simulink model "askisi3"  (R2021a)
settings: Solver=VariableStepAuto  StartTime=0.0  StopTime=1  RelTol=1e-3
libraries: spsCurrentMeasurementLib x3, spsVoltageMeasurementLib x3, spsRMSLib x2, spsAsynchronousMachineSIUnitsLib x1, spsNeutralLib x1, spsThreePhaseProgrammableVoltageSourceLib x1, spspowerguiLib x1
settings Model: Creator=up1053646  LastModifiedBy=up1053646

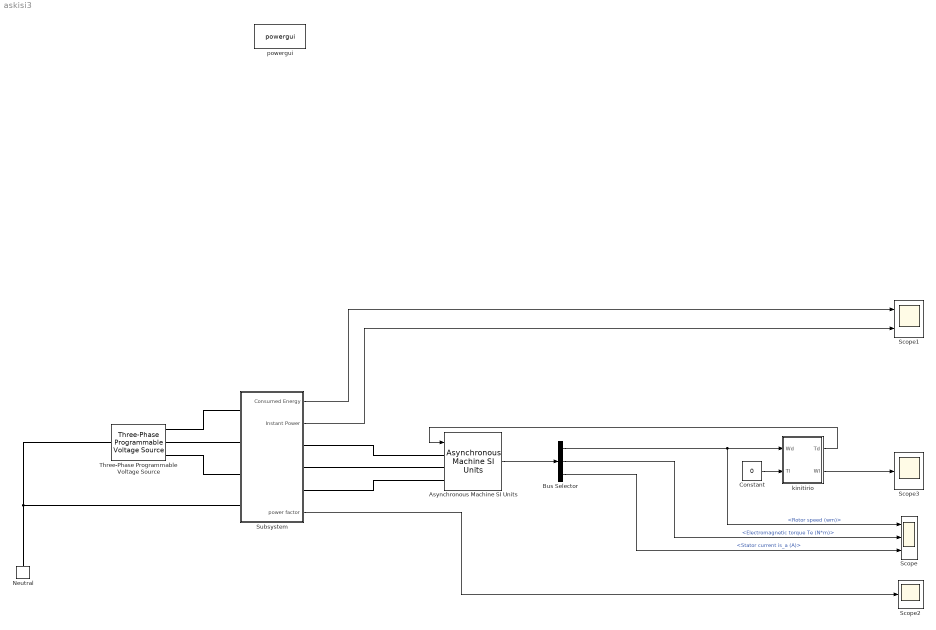
== system askisi3 ==
  Asynchronous Machine SI Units : spsAsynchronousMachineSIUnitsLib/Asynchronous Machine SI Units  RotorType=Squirrel-cage  PresetModel="15:  5.4 HP (4KW)   400 V  50Hz 1430 RPM"  MechanicalLoad=Torque Tm  ShowDetailedParameters=on  ReferenceFrame=Stationary  Units=SI  MeasurementBus=off  NominalParameters=[4000 400 50]  VoltageRatio=1  Stator=[1.405 0.005839]  Rotor=[1.395 0.005839]  Cage1=[0.4155 0.002066]  Cage2=[0.4168 0.0003495]  Lm=0.1722  Mechanical=[0.0131 0.002985 2]  PolePairs=2  InitialConditions=[1 0 0 0 0 0 0 0]  SimulateSaturation=off  Saturation=[14.03593122, 27.81365428, 53.79336849, 72.68890987, 97.98006896, 148.6815601, 215.7428561, 302.9841135, 428.7778367 ; 230, 322, 414, 460, 506, 552, 598, 644, 690]  LoadFlowParameters=1492000  TsPowergui=0  TsBlock=-1  IterativeModel=Trapezoidal non iterative  IterativeDiscreteModel=Trapezoidal non iterative  Pmec=1.492e+006
  Bus Selector : BusSelector  OutputSignals=Mechanical.Rotor speed (wm),Mechanical.Electromagnetic torque Te (N*m),Stator measurements.Stator current is_a (A)
  Constant : Constant  Value=0
  Neutral : spsNeutralLib/Neutral  LConnTagsString=a  NodeNumber=10
      settings: AttributesFormatString=node %<NodeNumber>  SourceProductBaseCode=PS
  Scope : Scope  NumInputPorts=3
  Scope1 : Scope  NumInputPorts=2
  Scope2 : Scope
  Scope3 : Scope
  Subsystem : Subsystem
      settings: PortSchema="{\"entries\":[{\"content\":{\"sides\":[{\"content\":{\"connectorIds\":[\"LConn1\",\"LConn2\",\"LConn3\",\"LConn4\"]},\"type\":\"ConnectorPlacement.EquallySpacedRectSide\",\"uuid\":\"32ddae11-412d-43d8-9429-097a82ad65a8\"},{\"content\":{\"connectorIds\":[\"Out1\",\"Out2\",\"RConn1\",\"RConn2\",\"RConn3\",\"Out3\"],\"side\":\"RIGHT\"},\"type\":\"ConnectorPlacement.EquallySpacedRectSide\",\"uuid\":\"05916abb-9d50-4f55-a81b-b25e6788eafb\"},{\"content\":{\"connectorIds\":[],\"side\":\"TOP\"},\"type\":\"ConnectorPlacement.EquallySpacedRectSide\",\"uuid\":\"ce3b48c4-ab88-427f-b81e-9245e7807eba\"}]},\"type\":\"ConnectorPlacement.EquallySpacedConnector\",\"uuid\":\"fa467998-3027-4402-b2bd-bbf2c58f6d7e\"}],\"packageUris\":[\"http://schema.mathworks.com/mf0/Connector/R2020b\"],\"version\":\"1.0\"}"
  Three-Phase Programmable Voltage Source : spsThreePhaseProgrammableVoltageSourceLib/Three-Phase Programmable Voltage Source  PositiveSequence="[380  0 50]"  VariationEntity=None  VariationType=Table of time-amplitude pairs  VariationTypeAlt=Step  VariationStep=0.5  VariationRate=10  VariationMagnitude=0.3  VariationFrequency=2  VariationTiming=[1 2]  VariationPhaseA=off  Amplitudes=[1 0.8 1.2 1.0]  TimeValues=[0 0.1 0.15 0.2]  HarmonicGeneration=off  HarmonicA=[3 0.2 -25 0]  HarmonicB=[2 0.15 35 2]  Timing="[0.05  3]"  BusType=swing  Pref=0  Qref=0  Qmin=-inf  Qmax=inf
  kinitirio : Subsystem  mask{kin=11000, bin=100, kout=20000, bout=1000, j=0.2, u=2, eff=1}
  powergui : spspowerguiLib/powergui  Priority=1  SimulationMode=Continuous  SampleTime=50e-6  frequency=60  Iterations=50  frequencyindice=50  Pbase=100e6  ErrMax=1e-4  UnitsV=kV  UnitsW=MW  buscounter=0  FunctionMessages=off  echomessages=off  EnableUseOfTLC=off  CurrentSourceSwitches=off  DisableSnubberDevices=off  DisableRonSwitches=off  DisableVfSwitches=off  DisplayEquations=off  AutomaticDiscreteSolvers=off  SolverType=Tustin/Backward Euler (TBE)  Interpol=off  ExternalGateDelay=off  methode=off  Ts=100  x0status=blocks  SPID=on  SwTol=0  HookPort=off  NonlinearTolerance=1e-4  nMaxIteration=100  ContinueOnMaxIteration=off  RestoreLinks=warning  ResistiveCurrentMeasurement=off  Frange=[0:2:500]  Ylog=off  Xlog=on  ShowGrid=off  save=off  variable=ZData  structure=0  ZoomFFT=off  StartTime=0.0  cycles=1  DisplayStyle=1  fundamental=60  FreqAxis=off  MaxFrequency=1000  frequencyindicesteady=1  RmsSteady=1  display=off
  wires:
  Bus Selector/1 -> kinitirio/1(Wd), Scope/1  "<Rotor speed (wm)>"
  Asynchronous Machine SI Units/1 -> Bus Selector/1
  Bus Selector/3 -> Scope/3  "<Stator current is_a (A)>"
  Bus Selector/2 -> Scope/2  "<Electromagnetic torque Te (N*m)>"
  Subsystem/3(power factor) -> Scope2/1
  Subsystem/1(Consumed Energy) -> Scope1/1
  Subsystem/2(Instant Power) -> Scope1/2
  kinitirio/2(Wl) -> Scope3/1
  Constant/1 -> kinitirio/2(Tl)
  kinitirio/1(Td) -> Asynchronous Machine SI Units/1
  connections:
  Subsystem/RConn1 -- Asynchronous Machine SI Units/LConn1
  Subsystem/RConn2 -- Asynchronous Machine SI Units/LConn2
  Subsystem/RConn3 -- Asynchronous Machine SI Units/LConn3
  Subsystem/LConn3 -- Three-Phase Programmable Voltage Source/RConn3
  Subsystem/LConn2 -- Three-Phase Programmable Voltage Source/RConn2
  Subsystem/LConn1 -- Three-Phase Programmable Voltage Source/RConn1
  Three-Phase Programmable Voltage Source/LConn1 -- Subsystem/LConn4 -- Neutral/LConn1

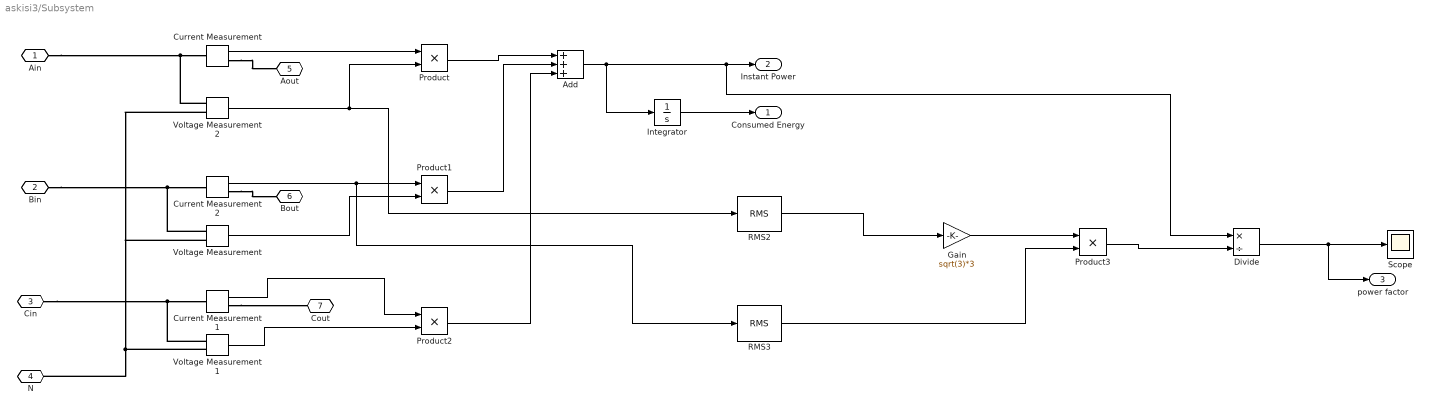
== system askisi3/Subsystem ==
  Add : Sum  Inputs=+++
  Current Measurement : spsCurrentMeasurementLib/Current Measurement  PhasorSimulation=off  OutputType=Complex  PSBequivalent=0
  Current Measurement1 : spsCurrentMeasurementLib/Current Measurement  PhasorSimulation=off  OutputType=Complex  PSBequivalent=0
  Current Measurement2 : spsCurrentMeasurementLib/Current Measurement  PhasorSimulation=off  OutputType=Complex  PSBequivalent=0
  Divide : Product  Inputs=*/
  Gain : Gain  Gain=sqrt(3)*3
  Integrator : Integrator
  Product{,1..3} (4 alike) : Product
  RMS2 : spsRMSLib/RMS  TrueRMS=on  Freq=50  RMSInit=120  Ts=0
  RMS3 : spsRMSLib/RMS  TrueRMS=on  Freq=50  RMSInit=120  Ts=0
  Scope : Scope
  Voltage Measurement : spsVoltageMeasurementLib/Voltage Measurement  PhasorSimulation=off  OutputType=Complex  PSBequivalent=0
  Voltage Measurement1 : spsVoltageMeasurementLib/Voltage Measurement  PhasorSimulation=off  OutputType=Complex  PSBequivalent=0
  Voltage Measurement2 : spsVoltageMeasurementLib/Voltage Measurement  PhasorSimulation=off  OutputType=Complex  PSBequivalent=0
  Ain : PMIOPort  Side=Left
  Bin : PMIOPort  Port=2  Side=Left
  Cin : PMIOPort  Port=3  Side=Left
  N : PMIOPort  Port=4  Side=Left
  Aout : PMIOPort  Port=5  Side=Right
  Bout : PMIOPort  Port=6  Side=Right
  Cout : PMIOPort  Port=7  Side=Right
  Consumed Energy : Outport
  Instant Power : Outport  Port=2
  power factor : Outport  Port=3
  wires:
  Current Measurement1/1 -> Product2/1
  Voltage Measurement1/1 -> Product2/2
  Voltage Measurement2/1 -> RMS2/1, Product/2
  Current Measurement2/1 -> RMS3/1, Product1/1
  Voltage Measurement/1 -> Product1/2
  Product/1 -> Add/1
  Product1/1 -> Add/2
  Product2/1 -> Add/3
  Add/1 -> Integrator/1, Divide/1, Instant Power/1
  Integrator/1 -> Consumed Energy/1
  Current Measurement/1 -> Product/1
  Gain/1 -> Product3/1
  RMS3/1 -> Product3/2
  Product3/1 -> Divide/2
  Divide/1 -> power factor/1, Scope/1
  RMS2/1 -> Gain/1
  connections:
  Ain/RConn1 -- Voltage Measurement2/LConn1 -- Current Measurement/LConn1
  Bin/RConn1 -- Voltage Measurement/LConn1 -- Current Measurement2/LConn1
  Cin/RConn1 -- Voltage Measurement1/LConn1 -- Current Measurement1/LConn1
  Voltage Measurement1/LConn2 -- Voltage Measurement2/LConn2 -- Voltage Measurement/LConn2 -- N/RConn1
  Current Measurement/RConn1 -- Aout/RConn1
  Current Measurement2/RConn1 -- Bout/RConn1
  Current Measurement1/RConn1 -- Cout/RConn1

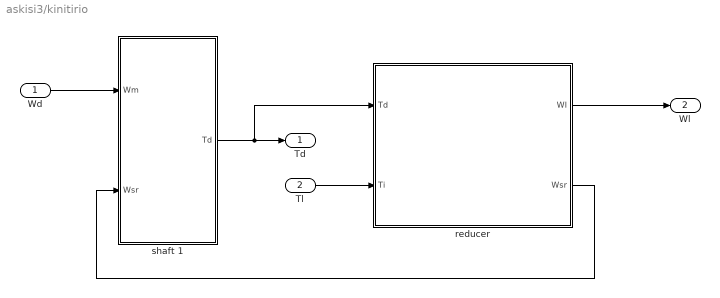
== system askisi3/kinitirio ==
  Wd : Inport
  Tl : Inport  Port=2
  reducer : Subsystem
  shaft 1 : Subsystem
  Td : Outport
  Wl : Outport  Port=2
  wires:
  Wd/1 -> shaft 1/1(Wm)
  shaft 1/1(Td) -> reducer/1(Td), Td/1
  reducer/2(Wsr) -> shaft 1/2(Wsr)
  reducer/1(WI) -> Wl/1
  Tl/1 -> reducer/2(Ti)

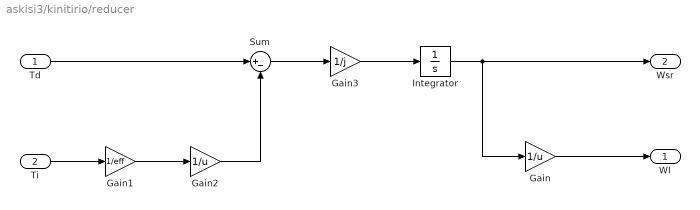
== system askisi3/kinitirio/reducer ==
  Td : Inport
  Ti : Inport  Port=2
  Gain : Gain  Gain=1/u
  Gain1 : Gain  Gain=1/eff
  Gain2 : Gain  Gain=1/u
  Gain3 : Gain  Gain=1/j
  Integrator : Integrator
  Sum : Sum  Inputs=|+-
  WI : Outport
  Wsr : Outport  Port=2
  wires:
  Ti/1 -> Gain1/1
  Gain1/1 -> Gain2/1
  Gain2/1 -> Sum/2
  Td/1 -> Sum/1
  Sum/1 -> Gain3/1
  Gain3/1 -> Integrator/1
  Integrator/1 -> Gain/1, Wsr/1
  Gain/1 -> WI/1

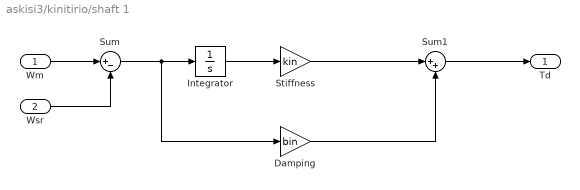
== system askisi3/kinitirio/shaft 1 ==
  Wm : Inport
  Wsr : Inport  Port=2
  Damping : Gain  Gain=bin
  Integrator : Integrator
  Stiffness : Gain  Gain=kin
  Sum : Sum  Inputs=|+-
  Sum1 : Sum  Inputs=|++
  Td : Outport
  wires:
  Wsr/1 -> Sum/2
  Wm/1 -> Sum/1
  Integrator/1 -> Stiffness/1
  Sum/1 -> Damping/1, Integrator/1
  Stiffness/1 -> Sum1/1
  Damping/1 -> Sum1/2
  Sum1/1 -> Td/1
